simulink model "PILEncoder"  (R2021a)
settings: Solver=FixedStepAuto  StartTime=0.0  StopTime=41.24  FixedStep=0.001  RelTol=1e-3  EnableMultiTasking=on
values from neighbouring files (symbols this model uses):
  den_lpf_d = den_lpf20    [Mainframe_init.m]    (also in load_autopilot.m)
  Emulated_FCC_IO_Delay = 7    [Mainframe_init.m]
  Enable_Gyros = 0    [Mainframe_init.m]
  Enable_INS = 0    [Mainframe_init.m]
  num_lpf_d = num_lpf20    [Mainframe_init.m]    (also in load_autopilot.m)
undefined symbols (not defined in the file or in its folder): act_dmp, act_omega, Actuator, Aerodynamics, aMode, Autopilot, AUX, c_b_WGS, c_be, c_flat, c_grav, c_h_geop0, c_h_geope, c_pa0, c_pe, c_r0, c_rot, c_rsma, c_Tmp0, d_siB_0, d_siB_max, d_siB_min, dd_siB_max, dd_siB_min, dev, DiscIntNeverNeededParam, e_pa, e_Tmp, Earth, fin_maxrate, flag_I_act_switch, flag_I_aero_switch, flag_I_flat, flag_I_gravity_switch, flag_I_rot, Flight_Logic, hcr, HIL_Data, JMMM_0, JMMM_e, JSPB_e, lat_0, lon_0, Main, Mass_Props, mB_0, mM_0, mM_e, pBII_0, pMPB, pNPB, propellant_kg, prp_FBPB, prp_mdot, prp_T, pSPB, pwm_output0, pwm_output1, qEG_0, qIB_0 ... (+30)
libraries: simulink x42, simulink_extras x24, aerolibcommonsys x4, px4lib x2, custom_blocks x1, dspstat3 x1, pil_lib x1, aerolibtransform2 x1, dspnetwork x1, aerolibnav x1
(part 9 of 16)

== system PILEncoder/Non-linear Flight Dynamic Model/GRM_Airframe/stream_flow/calc_stream_flow/velocity_vector_transformation/cross_product ==
  note: Outputs [size]:
      |
      | r1 x r2  [3x1]
  note: Inputs [size]:
      |
      | r1 [3x1]
      | r2 [3x1]
  r1 : Inport
  r2 : Inport  Port=2
  Demux2 : Demux  Outputs=[1;1;1]
      settings: DisplayOption=none
  Demux3 : Demux  Outputs=[1;1;1]
      settings: DisplayOption=none
  Product{2..7} (6 alike) : Product  InputSameDT=on  RndMeth=Zero  SaturateOnIntegerOverflow=on  OutDataTypeStr=Inherit: Same as first input
  Sum : Sum  Inputs=+-  InputSameDT=on  SaturateOnIntegerOverflow=on  OutDataTypeStr=Inherit: Same as first input
  Sum1 : Sum  Inputs=+-  InputSameDT=on  SaturateOnIntegerOverflow=on  OutDataTypeStr=Inherit: Same as first input
  Sum2 : Sum  Inputs=+-  InputSameDT=on  SaturateOnIntegerOverflow=on  OutDataTypeStr=Inherit: Same as first input
  Vector Concatenate : Concatenate  NumInputs=3  Mode=Multidimensional array
  r1_x_r2 : Outport  PortDimensions=[3,1]  VectorParamsAs1DForOutWhenUnconnected=off
  wires:
  Demux2/2 -> Product2/1, Product7/1
  Demux3/3 -> Product5/2, Product2/2
  Demux3/2 -> Product6/2, Product3/2
  Demux2/3 -> Product3/1, Product4/1
  Demux3/1 -> Product7/2, Product4/2
  Demux2/1 -> Product6/1, Product5/1
  Product2/1 -> Sum/1
  Product3/1 -> Sum/2
  Product4/1 -> Sum1/1
  Product5/1 -> Sum1/2
  Product6/1 -> Sum2/1
  Product7/1 -> Sum2/2
  Sum/1 -> Vector Concatenate/1
  Sum1/1 -> Vector Concatenate/2
  Sum2/1 -> Vector Concatenate/3
  r1/1 -> Demux2/1
  r2/1 -> Demux3/1
  Vector Concatenate/1 -> r1_x_r2/1

== system PILEncoder/Non-linear Flight Dynamic Model/GRM_Airframe/weight_and_balance/moi/moi_coordinate_transformation/3_rot_mat ==
  wi1 : Inport
  wi2 : Inport  Port=2
  wi3 : Inport  Port=3
  1. Rotation x-Achse : Subsystem
  1. Rotation y-Achse : Subsystem
  1. Rotation z-Achse : Subsystem
  2. Rotation x-Achse : Subsystem
  2. Rotation y-Achse : Subsystem
  2. Rotation z-Achse : Subsystem
  3. Rotation : Product  Inputs=***  Multiplication=Matrix(*)
  3. Rotation x-Achse : Subsystem
  3. Rotation y-Achse : Subsystem
  3. Rotation z-Achse : Subsystem
  Constant : Constant  Value=rot_1
  Constant1 : Constant  Value=rot_2
  Constant2 : Constant  Value=rot_3
  Multiport Switch : MultiPortSwitch
  Multiport Switch1 : MultiPortSwitch
  Multiport Switch2 : MultiPortSwitch
  T12 : Outport  VectorParamsAs1DForOutWhenUnconnected=off
  wires:
  Multiport Switch2/1 -> 3. Rotation/1
  Multiport Switch1/1 -> 3. Rotation/2
  Multiport Switch/1 -> 3. Rotation/3
  wi3/1 -> 3. Rotation x-Achse/1(alpha3), 3. Rotation z-Achse/1(alpha3), 3. Rotation y-Achse/1(alpha3)
  wi1/1 -> 1. Rotation z-Achse/1(alpha1), 1. Rotation y-Achse/1(alpha1), 1. Rotation x-Achse/1(alpha1)
  wi2/1 -> 2. Rotation z-Achse/1(alpha2), 2. Rotation y-Achse/1(alpha2), 2. Rotation x-Achse/1(alpha2)
  3. Rotation z-Achse/1(3Rot_Matrix_z) -> Multiport Switch2/4
  Constant/1 -> Multiport Switch/1
  1. Rotation x-Achse/1(1Rot_Matrix_x) -> Multiport Switch/2
  Constant1/1 -> Multiport Switch1/1
  1. Rotation y-Achse/1(1Rot_Matrix_y) -> Multiport Switch/3
  1. Rotation z-Achse/1(1Rot_Matrix_z) -> Multiport Switch/4
  Constant2/1 -> Multiport Switch2/1
  3. Rotation/1 -> T12/1  "T12"
  2. Rotation x-Achse/1(2Rot_Matrix_x) -> Multiport Switch1/2
  2. Rotation y-Achse/1(2Rot_Matrix_y) -> Multiport Switch1/3
  2. Rotation z-Achse/1(2Rot_Matrix_z) -> Multiport Switch1/4
  3. Rotation y-Achse/1(3Rot_Matrix_y) -> Multiport Switch2/3
  3. Rotation x-Achse/1(3Rot_Matrix_x) -> Multiport Switch2/2

== system PILEncoder/Non-linear Flight Dynamic Model/GRM_Airframe/weight_and_balance/moi/steiners_theorem_missile/create_deviation_matrix ==
  pBXB : Inport
  Add : Sum
  Add4 : Sum
  Add5 : Sum
  Demux : Demux  Outputs=3
  Gain : Gain  Gain=-1
  Gain1 : Gain  Gain=-1
  Gain3 : Gain  Gain=-1
  Product{1..6} (6 alike) : Product
  Vector Concatenate1 : Concatenate  NumInputs=3  Mode=Multidimensional array  ConcatenateDimension=2
  Vector Concatenate6 : Concatenate  NumInputs=3
  Vector Concatenate7 : Concatenate  NumInputs=3
  Vector Concatenate8 : Concatenate  NumInputs=3
  T_deviation : Outport  VectorParamsAs1DForOutWhenUnconnected=off
  wires:
  Add4/1 -> Vector Concatenate8/3
  Vector Concatenate6/1 -> Vector Concatenate1/1
  Vector Concatenate7/1 -> Vector Concatenate1/2
  Demux/1 -> Product3/1, Product4/1, Product5/2, Product5/1  "a"
  Demux/3 -> Product6/2, Product4/2, Product2/1, Product2/2  "c"
  Gain/1 -> Vector Concatenate7/1, Vector Concatenate6/2
  Gain3/1 -> Vector Concatenate8/2, Vector Concatenate7/3
  Vector Concatenate1/1 -> T_deviation/1
  Demux/2 -> Product3/2, Product1/2, Product1/1, Product6/1  "b"
  Add5/1 -> Vector Concatenate7/2
  Product6/1 -> Gain3/1
  Add/1 -> Vector Concatenate6/1
  Product1/1 -> Add5/1, Add/1
  Product5/1 -> Add4/2, Add5/2
  Product2/1 -> Add4/1, Add/2
  Gain1/1 -> Vector Concatenate8/1, Vector Concatenate6/3
  Product4/1 -> Gain1/1
  Product3/1 -> Gain/1
  Vector Concatenate8/1 -> Vector Concatenate1/3
  pBXB/1 -> Demux/1

== system PILEncoder/Non-linear Flight Dynamic Model/GRM_Airframe/weight_and_balance/moi/steiners_theorem_motor/create_deviation_matrix1 ==
  pBXB : Inport
  Add : Sum
  Add4 : Sum
  Add5 : Sum
  Demux : Demux  Outputs=3
  Gain : Gain  Gain=-1
  Gain1 : Gain  Gain=-1
  Gain3 : Gain  Gain=-1
  Product{1..6} (6 alike) : Product
  Vector Concatenate1 : Concatenate  NumInputs=3  Mode=Multidimensional array  ConcatenateDimension=2
  Vector Concatenate6 : Concatenate  NumInputs=3
  Vector Concatenate7 : Concatenate  NumInputs=3
  Vector Concatenate8 : Concatenate  NumInputs=3
  T_deviation : Outport  VectorParamsAs1DForOutWhenUnconnected=off
  wires:
  pBXB/1 -> Demux/1
  Vector Concatenate8/1 -> Vector Concatenate1/3
  Product3/1 -> Gain/1
  Product4/1 -> Gain1/1
  Gain1/1 -> Vector Concatenate6/3, Vector Concatenate8/1
  Product2/1 -> Add/2, Add4/1
  Product5/1 -> Add5/2, Add4/2
  Product1/1 -> Add/1, Add5/1
  Add/1 -> Vector Concatenate6/1
  Product6/1 -> Gain3/1
  Add5/1 -> Vector Concatenate7/2
  Demux/2 -> Product6/1, Product1/1, Product1/2, Product3/2  "b"
  Vector Concatenate1/1 -> T_deviation/1
  Gain3/1 -> Vector Concatenate7/3, Vector Concatenate8/2
  Gain/1 -> Vector Concatenate6/2, Vector Concatenate7/1
  Demux/3 -> Product2/2, Product2/1, Product4/2, Product6/2  "c"
  Demux/1 -> Product5/1, Product5/2, Product4/1, Product3/1  "a"
  Vector Concatenate7/1 -> Vector Concatenate1/2
  Vector Concatenate6/1 -> Vector Concatenate1/1
  Add4/1 -> Vector Concatenate8/3

== system PILEncoder/Non-linear Flight Dynamic Model/Subsystem1/Extract States/Assemble_States_Bus1/Three-axis Inertial Measurement Unit3/Acceleration Conversion ==
  acceleration : Inport  Unit=m/s^2
  Unit Conversion : UnitConversion
  inherit : Outport  VectorParamsAs1DForOutWhenUnconnected=off
  wires:
  acceleration/1 -> Unit Conversion/1
  Unit Conversion/1 -> inherit/1

== system PILEncoder/Non-linear Flight Dynamic Model/Subsystem1/Extract States/Assemble_States_Bus1/Three-axis Inertial Measurement Unit3/Three-axis Accelerometer ==
  Ab : Inport  Unit=m/s^2  PortDimensions=3
  p q r : Inport  Port=2  Unit=rad/s
  pdot qdot rdot : Inport  Port=3  Unit=rad/s^2
  CG : Inport  Port=4  Unit=m  PortDimensions=3
  g : Inport  Port=5  Unit=m/s^2
  Disallow CGS : UnitConfiguration  UnitSystemsStr=English,SI,SI (extended)  AllowAllUnitSystems=off
  Dynamics : Subsystem
  Gain : Gain  Gain=[1 -1 1]  SaturateOnIntegerOverflow=on  OutDataTypeStr=Inherit: Same as input  ParamDataTypeStr=Inherit: Same as input
  Measurement bias : Constant  Value=a_bias
  Product : Product  Multiplication=Matrix(*)  SaturateOnIntegerOverflow=on  OutDataTypeStr=Inherit: Same as first input
  Random bias : aerolibcommonsys/Tunable White Noise  pwr=a_pow  Ts=0.1  seed=a_seeds
      settings: SourceProductBaseCode=AE
  Reshape1 : Reshape
  Saturation : Saturate  UpperLimit=a_sath  LowerLimit=a_satl
  Scale factors & Cross-coupling errors : Constant  Value=a_sf_cc
  Sum : Sum  Inputs=+-++  SaturateOnIntegerOverflow=on
  Sum1 : Sum  Inputs=|++  SaturateOnIntegerOverflow=on
  Sum4 : Sum  Inputs=++|  SaturateOnIntegerOverflow=on
  Sum7 : Sum  Inputs=|+-  SaturateOnIntegerOverflow=on
  Zero-Order Hold{,1..4} (5 alike) : Gain  SaturateOnIntegerOverflow=on  OutDataTypeStr=Inherit: Same as input  ParamDataTypeStr=Inherit: Same as input
  w x (w x d) : Subsystem
  wdot x d : Subsystem  mask(CrossProduct){aMode=aMode}
      mask help: shared_aeroblks:sharedaeroblkutil:blockCrossProductDesc
      mask init:
      | if aerosharedtest(gcb)
      |     aerosharedicon('shared');
      | else
      |     sharedautoicon('shared');
      | end
      mask Help: eval('if license(''test'',''Aerospace_Blockset'')aerosharedhelp(''threebythree_cross_product'');elseif license(''test'',''Powertrain_Blockset'')sharedautohelp(''threebythree_cross_product'');end')
      mask Display:
      | text(.5,.5,'Cross\nProduct\nC = AxB', ...
      | 	'HorizontalAlignment','Center',...
      | 	'VerticalAlignment','middle')
  wl_ins : Constant  Value=acc
  Ameas : Outport  Unit=m/s^2  PortDimensions=3  VectorParamsAs1DForOutWhenUnconnected=off
  wires:
  Zero-Order Hold4/1 -> Sum7/1
  Zero-Order Hold3/1 -> wdot x d/1(A)
  Zero-Order Hold/1 -> w x (w x d)/1("p q r ")
  Zero-Order Hold2/1 -> Sum/2
  Zero-Order Hold1/1 -> Sum/1
  g/1 -> Zero-Order Hold2/1
  Gain/1 -> wdot x d/2(B), w x (w x d)/2(distance)
  wl_ins/1 -> Sum7/2
  Sum7/1 -> Gain/1
  Dynamics/1("sp_f ") -> Sum1/1
  Sum4/1 -> Dynamics/1(sp_f)
  Sum1/1 -> Saturation/1
  w x (w x d)/1(w x ( w x d)) -> Sum/3
  Ab/1 -> Zero-Order Hold1/1
  Reshape1/1 -> Sum4/1
  Measurement bias/1 -> Sum4/2
  Product/1 -> Reshape1/1
  CG/1 -> Zero-Order Hold4/1
  pdot qdot rdot/1 -> Zero-Order Hold3/1
  p q r/1 -> Zero-Order Hold/1
  Sum/1 -> Product/2
  wdot x d/1(C) -> Sum/4
  Scale factors & Cross-coupling errors/1 -> Product/1
  Random bias/1 -> Sum1/2
  Saturation/1 -> Ameas/1

== system PILEncoder/Non-linear Flight Dynamic Model/Subsystem1/Extract States/Assemble_States_Bus1/Three-axis Inertial Measurement Unit3/Three-axis Gyroscope ==
  p q r : Inport  Unit=rad/s  PortDimensions=3
  G's : Inport  Port=2  Unit=gn  PortDimensions=3
  Disallow CGS : UnitConfiguration  UnitSystemsStr=English,SI,SI (extended)  AllowAllUnitSystems=off
  Dynamics : Subsystem
  Measurement bias : Constant  Value=g_bias
  Product : Product  Multiplication=Matrix(*)  SaturateOnIntegerOverflow=on  OutDataTypeStr=Inherit: Same as first input
  Product1 : Product  SaturateOnIntegerOverflow=on  OutDataTypeStr=Inherit: Same as first input
  Random bias : aerolibcommonsys/Tunable White Noise  pwr=g_pow  Ts=0.1  seed=g_seeds
      settings: SourceProductBaseCode=AE
  Saturation : Saturate  UpperLimit=g_sath  LowerLimit=g_satl
  "Scale factors & Cross-coupling errors " : Constant  Value=g_sf_cc
  Sum1 : Sum  Inputs=|++  SaturateOnIntegerOverflow=on
  Sum4 : Sum  Inputs=+++  SaturateOnIntegerOverflow=on
  Zero-Order Hold : Gain  SaturateOnIntegerOverflow=on  OutDataTypeStr=Inherit: Same as input  ParamDataTypeStr=Inherit: Same as input
  Zero-Order Hold1 : Gain  SaturateOnIntegerOverflow=on  OutDataTypeStr=Inherit: Same as input  ParamDataTypeStr=Inherit: Same as input
  g-sensitive bias : Constant  Value=g_sen
  (p q r)_meas : Outport  Unit=rad/s  PortDimensions=3  VectorParamsAs1DForOutWhenUnconnected=off
  wires:
  Zero-Order Hold1/1 -> Product1/1
  Zero-Order Hold/1 -> Product/2
  Product1/1 -> Sum4/3
  Dynamics/1("p q r ") -> Sum1/1
  G's/1 -> Zero-Order Hold1/1
  Sum1/1 -> Saturation/1
  g-sensitive bias/1 -> Product1/2
  p q r/1 -> Zero-Order Hold/1
  Saturation/1 -> (p q r)_meas/1
  Random bias/1 -> Sum1/2
  "Scale factors & Cross-coupling errors "/1 -> Product/1
  Sum4/1 -> Dynamics/1(p q r)
  Product/1 -> Sum4/1
  Measurement bias/1 -> Sum4/2

== system PILEncoder/Non-linear Flight Dynamic Model/Subsystem1/GRM_Airframe/aerodynamics/aerodynamic_via_lookup/calc_aero_coefficients ==
  dela_deg : Inport
  dele_deg : Inport  Port=2
  delr_deg : Inport  Port=3
  pBIB_star_rps : Inport  Port=4
  qBIB_star_rps : Inport  Port=5
  rBIB_star_rps : Inport  Port=6
  alB_deg : Inport  Port=7
  beB_deg : Inport  Port=8
  CLL_TLU : Subsystem
  CLM_TLU : Subsystem
  CLN_TLU : Subsystem
  CX_TLU : Subsystem
  CY_TLU : Subsystem
  CZ_TLU : Subsystem
  alB_deg D{1..5} (5 alike) : InportShadow  Port=7
  beB_deg D{1..5} (5 alike) : InportShadow  Port=8
  dela_deg D{1..6} (6 alike) : InportShadow
  dele_deg D{1..4} (4 alike) : InportShadow  Port=2
  delr_deg D{1..5} (5 alike) : InportShadow  Port=3
  Cx : Outport  VectorParamsAs1DForOutWhenUnconnected=off
  Cy : Outport  Port=2  VectorParamsAs1DForOutWhenUnconnected=off
  Cz : Outport  Port=3  VectorParamsAs1DForOutWhenUnconnected=off
  Cl : Outport  Port=4  VectorParamsAs1DForOutWhenUnconnected=off
  Cm : Outport  Port=5  VectorParamsAs1DForOutWhenUnconnected=off
  Cn : Outport  Port=6  VectorParamsAs1DForOutWhenUnconnected=off
  wires:
  CX_TLU/1(CX) -> Cx/1
  alB_deg/1 -> CX_TLU/1(alpha_deg)
  beB_deg/1 -> CX_TLU/2(beta_deg)
  dele_deg/1 -> CX_TLU/3(dele_deg)
  dela_deg/1 -> CX_TLU/4(dela_deg)
  CY_TLU/1(CY) -> Cy/1
  beB_deg D1/1 -> CY_TLU/2(beta_deg)
  alB_deg D1/1 -> CY_TLU/1(alpha_deg)
  delr_deg/1 -> CX_TLU/5(delr_deg)
  CZ_TLU/1(CZ) -> Cz/1
  CLL_TLU/1(CLL) -> Cl/1
  CLM_TLU/1(CLM) -> Cm/1
  CLN_TLU/1(CLN) -> Cn/1
  pBIB_star_rps/1 -> CLL_TLU/6(p_ND_rps)
  qBIB_star_rps/1 -> CLM_TLU/6(q_ND_rps)
  rBIB_star_rps/1 -> CLN_TLU/6(r_ND_rps)
  alB_deg D2/1 -> CZ_TLU/1(alpha_deg)
  beB_deg D2/1 -> CZ_TLU/2(beta_deg)
  dele_deg D1/1 -> CY_TLU/3(dele_deg)
  dela_deg D1/1 -> CY_TLU/4(dela_deg)
  delr_deg D1/1 -> CY_TLU/5(delr_deg)
  dele_deg D2/1 -> CZ_TLU/3(dele_deg)
  dela_deg D2/1 -> CZ_TLU/4(dela_deg)
  delr_deg D2/1 -> CZ_TLU/5(delr_deg)
  dela_deg D3/1 -> CLN_TLU/3(dele_deg)
  dela_deg D4/1 -> CLN_TLU/4(dela_deg)
  delr_deg D3/1 -> CLN_TLU/5(delr_deg)
  alB_deg D5/1 -> CLN_TLU/1(alpha_deg)
  alB_deg D4/1 -> CLM_TLU/1(alpha_deg)
  alB_deg D3/1 -> CLL_TLU/1(alpha_deg)
  beB_deg D3/1 -> CLL_TLU/2(beta_deg)
  beB_deg D4/1 -> CLM_TLU/2(beta_deg)
  beB_deg D5/1 -> CLN_TLU/2(beta_deg)
  dele_deg D3/1 -> CLL_TLU/3(dele_deg)
  dele_deg D4/1 -> CLM_TLU/3(dele_deg)
  dela_deg D5/1 -> CLL_TLU/4(dela_deg)
  dela_deg D6/1 -> CLM_TLU/4(dela_deg)
  delr_deg D4/1 -> CLL_TLU/5(delr_deg)
  delr_deg D5/1 -> CLM_TLU/5(delr_deg)

== system PILEncoder/Non-linear Flight Dynamic Model/Subsystem1/GRM_Airframe/aerodynamics/aerodynamic_via_lookup/calc_aero_for_mom ==
  hBE : Inport
  pBPB : Inport  Port=2
  qdynB : Inport  Port=3
  Cx : Inport  Port=4
  Cy : Inport  Port=5
  Cz : Inport  Port=6
  Cl : Inport  Port=7
  Cm : Inport  Port=8
  Cn : Inport  Port=9
  Add : Sum
  Constant1 : Constant  Value=Aerodynamics.lref
      settings: AttributesFormatString=%<Value>
  Constant2 : Constant  Value=Aerodynamics.sref
      settings: AttributesFormatString=%<Value>
  Product : Product
  Product1 : Product  Inputs=3
  Product2 : Product
  Subtract : Sum  Inputs=+-
  Vector Concatenate1 : Concatenate  NumInputs=3
  Vector Concatenate2 : Concatenate  NumInputs=3
  create_pAPB : Subsystem
  cross_product : Subsystem
      mask help: cross product r3 = r1 x r2
      mask Help:
      | Name:
      | 
      |     cross_product
      | 
      | Description:
      | 
      |     This block implements the cross product r3 = r1 x r2.
      | 
      | Inputs  [size] [data type] [unit]:
      | 
      |     vector 1  [3] [double] [-]
      |     vector 2  [3] [double] [-]
      | 
      | Outputs  [size] [data type] [unit]:
      | 
      |     resulting vector  [3] [double] [-]
      mask Display: disp(' r3 = r1 x r2')
  launch_rail : Subsystem
  launch_rail1 : Subsystem
  FBAB : Outport  VectorParamsAs1DForOutWhenUnconnected=off
  MBAB : Outport  Port=2  VectorParamsAs1DForOutWhenUnconnected=off
  wires:
  Cy/1 -> Vector Concatenate2/2
  Cm/1 -> Vector Concatenate1/2
  Cz/1 -> Vector Concatenate2/3
  Cx/1 -> Vector Concatenate2/1
  Cl/1 -> Vector Concatenate1/1
  Cn/1 -> Vector Concatenate1/3
  qdynB/1 -> Product2/2
  Vector Concatenate1/1 -> Product1/2
  Vector Concatenate2/1 -> Product/1
  pBPB/1 -> Subtract/2
  Product/1 -> launch_rail/2(FBAB_c), cross_product/2(r2)  "FBAB"
  Product1/1 -> Add/2  "MBAB"
  Add/1 -> launch_rail1/2(MBAB_c)  "MBAB"
  Constant1/1 -> Product1/3
  Constant2/1 -> Product2/1
  Product2/1 -> Product1/1, Product/2
  cross_product/1(r1_x_r2) -> Add/1
  hBE/1 -> launch_rail1/1(hBE), launch_rail/1(hBE)
  launch_rail1/1(MBAB) -> MBAB/1
  launch_rail/1(FBAB) -> FBAB/1
  Subtract/1 -> cross_product/1(r1)  "pBAB"
  create_pAPB/1(pAPB) -> Subtract/1

== system PILEncoder/Non-linear Flight Dynamic Model/Subsystem1/GRM_Airframe/environment/WGS84_Gravitation/WGS84_2_ECEF ==
  h : Inport
  lon : Inport  Port=2
  lat : Inport  Port=3
  Add1 : Sum  Inputs=+-
  Add2 : Sum
  Add3 : Sum
  Constant : Constant
  Divide : Product  Inputs=***
  Divide1 : Product  Inputs=***
  Divide2 : Product  Inputs=**
  Divide3 : Product  Inputs=**
  Divide4 : Product  Inputs=**
  Mux : Mux  Inputs=3
  Trigonometric Function : Trigonometry
  Trigonometric Function1 : Trigonometry  Operator=cos
  Trigonometric Function2 : Trigonometry
  Trigonometric Function3 : Trigonometry  Operator=cos
  "WGS84 Transformation Parameter " : Subsystem
  pE : Outport  VectorParamsAs1DForOutWhenUnconnected=off
  wires:
  Divide1/1 -> Mux/2  "y_ECEF"
  Add2/1 -> Divide4/1
  Divide/1 -> Mux/1  "x_ECEF"
  lat/1 -> "WGS84 Transformation Parameter "/1(phi), Trigonometric Function3/1, Trigonometric Function2/1
  Divide2/1 -> Add1/2
  Divide3/1 -> Add2/2  "N(1-e^2)"
  Constant/1 -> Add1/1
  Add1/1 -> Divide3/2
  Divide4/1 -> Mux/3  "z_ECEF"
  "WGS84 Transformation Parameter "/1(N) -> Add3/2, Divide3/1
  "WGS84 Transformation Parameter "/2(e) -> Divide2/2, Divide2/1
  h/1 -> Add2/1, Add3/1
  Trigonometric Function1/1 -> Divide/2  "cos(lambda)"
  Trigonometric Function3/1 -> Divide1/3, Divide/3  "cos(phi)"
  Mux/1 -> pE/1  "pE"
  lon/1 -> Trigonometric Function1/1, Trigonometric Function/1
  Add3/1 -> Divide1/1, Divide/1
  Trigonometric Function2/1 -> Divide4/2  "sin(phi)"
  Trigonometric Function/1 -> Divide1/2  "sin(lambda)"

== system PILEncoder/Non-linear Flight Dynamic Model/Subsystem1/GRM_Airframe/environment/atmosphere_static_ISO_2533/density ==
  Tmp : Inport
  pa : Inport  Port=2
  Divide : Product  Inputs=/*/
  specific_gas_constant : Constant  Value=sgc
  rho : Outport  VectorParamsAs1DForOutWhenUnconnected=off
  wires:
  Tmp/1 -> Divide/1
  Divide/1 -> rho/1  "rho"
  pa/1 -> Divide/2
  specific_gas_constant/1 -> Divide/3

== system PILEncoder/Non-linear Flight Dynamic Model/Subsystem1/GRM_Airframe/environment/atmosphere_static_ISO_2533/geopot_height ==
  hBE : Inport
  Add : Sum
  Divide : Product  Inputs=*/*
  mean_earth_radius : Constant  Value=mean_earth_radius
  h_geop : Outport  VectorParamsAs1DForOutWhenUnconnected=off
  wires:
  mean_earth_radius/1 -> Divide/3, Add/2
  Divide/1 -> h_geop/1  "h_geop"
  hBE/1 -> Add/1, Divide/1
  Add/1 -> Divide/2

== system PILEncoder/Non-linear Flight Dynamic Model/Subsystem1/GRM_Airframe/environment/atmosphere_static_ISO_2533/speed_of_sound ==
  Tmp : Inport
  Product : Product  Inputs=3
  Sqrt : Sqrt  SaturateOnIntegerOverflow=on
  heat_capacity_ratio : Constant  Value=hcr
  specific_gas_constant : Constant  Value=sgc
  sos : Outport  VectorParamsAs1DForOutWhenUnconnected=off
  wires:
  Sqrt/1 -> sos/1  "sos"
  Tmp/1 -> Product/3
  Product/1 -> Sqrt/1
  heat_capacity_ratio/1 -> Product/2
  specific_gas_constant/1 -> Product/1

== system PILEncoder/Non-linear Flight Dynamic Model/Subsystem1/GRM_Airframe/environment/atmosphere_static_ISO_2533/tmp_and_pressure_ISO_2533 ==
  h_geop : Inport
  e_Tmp : Inport  Port=2
  e_pa : Inport  Port=3
  Subtract1 : Sum
  Subtract2 : Sum
  Tmp_norm_msl : Constant  Value=c_Tmp0
  geopotential_height_ref : Constant  Value=c_h_geop0
  pa_norm_msl : Constant  Value=c_pa0
  static_Temperature : Subsystem
  static_pressure : Subsystem
  Tmp : Outport  VectorParamsAs1DForOutWhenUnconnected=off
  pa : Outport  Port=2  VectorParamsAs1DForOutWhenUnconnected=off
  wires:
  h_geop/1 -> static_pressure/2(h_geop), static_Temperature/2(h_geop)
  Subtract2/1 -> static_pressure/4(pa_ref)  "pa_ref"
  pa_norm_msl/1 -> Subtract2/2
  Subtract1/1 -> static_pressure/3(Tmp_ref), static_Temperature/1(Tmp_ref)  "Tmp_ref"
  static_pressure/1(pa) -> pa/1
  e_pa/1 -> Subtract2/1
  static_Temperature/1(Tmp) -> Tmp/1
  e_Tmp/1 -> Subtract1/1
  geopotential_height_ref/1 -> static_pressure/1(h_geop_ref), static_Temperature/3(h_geop_ref)  "h_geop_ref"
  Tmp_norm_msl/1 -> Subtract1/2

== system PILEncoder/Non-linear Flight Dynamic Model/Subsystem1/GRM_Airframe/gravity/launch_rail/initial_altitude ==
  Constant : Constant  Value=pBII_0
  Constant2 : Constant  Value=flag_I_flat
  Demux : Demux  Outputs=3
  Gain : Gain  Gain=-1
  Switch1 : Switch  Criteria=u2 > Threshold
  Terminator{,1..3} (4 alike) : Terminator
  trafo_E_to_geodetic : Subsystem  mask(Transformation der ECEF Position in geodätische Größen){}
      mask help: Dieser Block transformiert die Position im ECEF KOS in die geodätische Länge, Breite und Höhe
      mask init:
      | [c_mue, c_rsma, c_flat] = init_transformations_earth;
      mask Help:
      | Name:
      | 
      |     trafo_E_to_geodetic
      | 
      | Beschreibung:
      | 
      |     Dieser Block transformiert die Position im ECEF KOS in die geodätische
      |     Länge, Breite und Höhe.
      | 
      | Inputs   [size]  [data type] [unit]:
      | 
      |     pBEE    [3] [double] [m]
      | 
      | Outputs  [size]  [data type] [unit]:
      | 
      |     long  [1] [double] [rad]
      |     lat   [1] [double] [rad]
      |     alt   [1] [double] [m]
      | 
      | Parameter
      | 
      |    c_rsma
      |    c_flat
  hBE_0 : Outport  VectorParamsAs1DForOutWhenUnconnected=off
  wires:
  Constant2/1 -> Switch1/2
  trafo_E_to_geodetic/3(alt) -> Switch1/3  "hBE_0"
  Demux/2 -> Terminator3/1
  Demux/3 -> Gain/1
  Gain/1 -> Switch1/1
  Demux/1 -> Terminator2/1
  trafo_E_to_geodetic/2(lat) -> Terminator1/1
  Constant/1 -> Demux/1, trafo_E_to_geodetic/1(pBEE)
  trafo_E_to_geodetic/1(lon) -> Terminator/1
  Switch1/1 -> hBE_0/1  "hBE_0"

== system PILEncoder/Non-linear Flight Dynamic Model/Subsystem1/GRM_Airframe/motion_kinematics/calc_motion_kinematics/calc_transformation_matrix ==
  qIE : Inport
  qEG : Inport  Port=2
  qIB : Inport  Port=3
  T12_from_q1 : Subsystem
      mask help: Transforms a quaternion into a Direction Cosine Matrix
      mask Help:
      | Name:
      | 
      |     T12_from_q12
      | 
      | Description:
      | 
      |     This block implements the transformation of a quaternion into the
      |     corresponding direction cosine matrix DCM.
      | 
      | Inputs  [size] [data type] [unit]:
      | 
      |     quaternion q12 [4] [double] [-]
      | 
      | Outputs  [size] [data type] [unit]:
      | 
      |     direction cosine matrix T12  [3x3] [double] [-]
      mask Display:
      | %port_label('input', 1, 'q12')
      | %port_label('output', 1, 'T12')
      | disp('q \rightarrow DCM','texmode','on')
  T12_from_q12 : Subsystem
      mask help: Transforms a quaternion into a Direction Cosine Matrix
      mask Help:
      | Name:
      | 
      |     T12_from_q12
      | 
      | Description:
      | 
      |     This block implements the transformation of a quaternion into the
      |     corresponding direction cosine matrix DCM.
      | 
      | Inputs  [size] [data type] [unit]:
      | 
      |     quaternion q12 [4] [double] [-]
      | 
      | Outputs  [size] [data type] [unit]:
      | 
      |     direction cosine matrix T12  [3x3] [double] [-]
      mask Display:
      | %port_label('input', 1, 'q12')
      | %port_label('output', 1, 'T12')
      | disp('q \rightarrow DCM','texmode','on')
  T12_from_q2 : Subsystem
      mask help: Transforms a quaternion into a Direction Cosine Matrix
      mask Help:
      | Name:
      | 
      |     T12_from_q12
      | 
      | Description:
      | 
      |     This block implements the transformation of a quaternion into the
      |     corresponding direction cosine matrix DCM.
      | 
      | Inputs  [size] [data type] [unit]:
      | 
      |     quaternion q12 [4] [double] [-]
      | 
      | Outputs  [size] [data type] [unit]:
      | 
      |     direction cosine matrix T12  [3x3] [double] [-]
      mask Display:
      | %port_label('input', 1, 'q12')
      | %port_label('output', 1, 'T12')
      | disp('q \rightarrow DCM','texmode','on')
  conjugate_quaternion : Subsystem
      mask help: conjugate a quaternion
      mask Help:
      | Name:
      | 
      |     conjugate_quaternion
      | 
      | Description:
      | 
      |     computes the conjugate quaternion
      | 
      | Inputs  [size] [data type] [unit]:
      | 
      |     quaternion q_2_1  [4] [double] [-]
      | 
      | Outputs  [size] [data type] [unit]:
      | 
      |     conjugated quaternion q_1_2  [4] [double] [-]
      mask Display: disp (' conj(q)')
  q31_from_q32_mul_q1 : Subsystem
      mask help: multiply two quaternions
      mask Help:
      | Name:
      | 
      |     q31_from_q32_mul_q21
      | 
      | Description:
      | 
      |     This block implements the multiplication of two quaternions according
      |     to q31=q32*q21.
      | 
      | Inputs  [size] [data type] [unit]:
      | 
      |     attitude quaternion q32  [4] [double] [-]
      |     attitude quaternion q21  [4] [double] [-]
      | 
      | Outputs  [size] [data type] [unit]:
      | 
      |     attitude quaternion q31  [4] [double] [-]
      mask Display:
      | port_label('input', 1, 'q32')
      | port_label('input', 2, 'q21')
      | port_label('output', 1, 'q31')
      | disp('q_{31} = q_{32} {\bf\cdot} q_{21}','texmode','on')
  q31_from_q32_mul_q2 : Subsystem
      mask help: multiply two quaternions
      mask Help:
      | Name:
      | 
      |     q31_from_q32_mul_q21
      | 
      | Description:
      | 
      |     This block implements the multiplication of two quaternions according
      |     to q31=q32*q21.
      | 
      | Inputs  [size] [data type] [unit]:
      | 
      |     attitude quaternion q32  [4] [double] [-]
      |     attitude quaternion q21  [4] [double] [-]
      | 
      | Outputs  [size] [data type] [unit]:
      | 
      |     attitude quaternion q31  [4] [double] [-]
      mask Display:
      | port_label('input', 1, 'q32')
      | port_label('input', 2, 'q21')
      | port_label('output', 1, 'q31')
      | disp('q_{31} = q_{32} {\bf\cdot} q_{21}','texmode','on')
  q31_from_q32_mul_q21 : Subsystem
      mask help: multiply two quaternions
      mask Help:
      | Name:
      | 
      |     q31_from_q32_mul_q21
      | 
      | Description:
      | 
      |     This block implements the multiplication of two quaternions according
      |     to q31=q32*q21.
      | 
      | Inputs  [size] [data type] [unit]:
      | 
      |     attitude quaternion q32  [4] [double] [-]
      |     attitude quaternion q21  [4] [double] [-]
      | 
      | Outputs  [size] [data type] [unit]:
      | 
      |     attitude quaternion q31  [4] [double] [-]
      mask Display:
      | port_label('input', 1, 'q32')
      | port_label('input', 2, 'q21')
      | port_label('output', 1, 'q31')
      | disp('q_{31} = q_{32} {\bf\cdot} q_{21}','texmode','on')
  TEB : Outport  VectorParamsAs1DForOutWhenUnconnected=off
  TGB : Outport  Port=2  VectorParamsAs1DForOutWhenUnconnected=off
  TIB : Outport  Port=3  VectorParamsAs1DForOutWhenUnconnected=off
  wires:
  T12_from_q2/1(T12) -> TGB/1  "TGB"
  q31_from_q32_mul_q21/1(q31) -> conjugate_quaternion/1(q)  "qIG"
  qIB/1 -> q31_from_q32_mul_q1/2(q21), T12_from_q12/1(q12)
  q31_from_q32_mul_q1/1(q31) -> T12_from_q2/1(q12), q31_from_q32_mul_q2/2(q21)  "qGB"
  qEG/1 -> q31_from_q32_mul_q21/2(q21), q31_from_q32_mul_q2/1(q32)
  T12_from_q1/1(T12) -> TEB/1  "TEB"
  conjugate_quaternion/1(q_conj) -> q31_from_q32_mul_q1/1(q32)  "qGI"
  qIE/1 -> q31_from_q32_mul_q21/1(q32)
  q31_from_q32_mul_q2/1(q31) -> T12_from_q1/1(q12)  "qEB"
  T12_from_q12/1(T12) -> TIB/1  "TIB"

== system PILEncoder/Non-linear Flight Dynamic Model/Subsystem1/GRM_Airframe/motion_kinematics/calc_motion_kinematics/earth_rotation ==
  lat : Inport
  lon : Inport  Port=2
  Gain : Gain
  Gain1 : Gain
  earth_rotation_rate : Subsystem
  quaternion_integration : Subsystem
  quaternion_integration1 : Subsystem
  transport_rate : Subsystem
  wIEE : Outport  VectorParamsAs1DForOutWhenUnconnected=off
  TIE : Outport  Port=2  VectorParamsAs1DForOutWhenUnconnected=off
  qIE : Outport  Port=3  VectorParamsAs1DForOutWhenUnconnected=off
  qEG : Outport  Port=4  VectorParamsAs1DForOutWhenUnconnected=off
  TEG : Outport  Port=5  VectorParamsAs1DForOutWhenUnconnected=off
  wEGG : Outport  Port=6  VectorParamsAs1DForOutWhenUnconnected=off
  wires:
  earth_rotation_rate/1(wIEE) -> wIEE/1, Gain/1
  Gain/1 -> quaternion_integration/1(wEIE)  "wEIE"
  quaternion_integration/1(qIE) -> qIE/1
  quaternion_integration/2(TIE) -> TIE/1
  lat/1 -> transport_rate/1(lat)
  lon/1 -> transport_rate/2(lon)
  transport_rate/1(wEGG) -> wEGG/1, Gain1/1
  Gain1/1 -> quaternion_integration1/1(wGEG)  "wGEG"
  quaternion_integration1/1(qEG) -> qEG/1
  quaternion_integration1/2(TEG) -> TEG/1

== system PILEncoder/Non-linear Flight Dynamic Model/Subsystem1/GRM_Airframe/propulsion/prp_uncertainty/3_rot_mat ==
  wi1 : Inport
  wi2 : Inport  Port=2
  wi3 : Inport  Port=3
  1. Rotation x-Achse : Subsystem
  1. Rotation y-Achse : Subsystem
  1. Rotation z-Achse : Subsystem
  2. Rotation x-Achse : Subsystem
  2. Rotation y-Achse : Subsystem
  2. Rotation z-Achse : Subsystem
  3. Rotation : Product  Inputs=***  Multiplication=Matrix(*)
  3. Rotation x-Achse : Subsystem
  3. Rotation y-Achse : Subsystem
  3. Rotation z-Achse : Subsystem
  Constant : Constant  Value=rot_1
  Constant1 : Constant  Value=rot_2
  Constant2 : Constant  Value=rot_3
  Multiport Switch : MultiPortSwitch
  Multiport Switch1 : MultiPortSwitch
  Multiport Switch2 : MultiPortSwitch
  T12 : Outport  VectorParamsAs1DForOutWhenUnconnected=off
  wires:
  Multiport Switch2/1 -> 3. Rotation/1
  Multiport Switch1/1 -> 3. Rotation/2
  Multiport Switch/1 -> 3. Rotation/3
  wi3/1 -> 3. Rotation x-Achse/1(alpha3), 3. Rotation z-Achse/1(alpha3), 3. Rotation y-Achse/1(alpha3)
  wi1/1 -> 1. Rotation z-Achse/1(alpha1), 1. Rotation y-Achse/1(alpha1), 1. Rotation x-Achse/1(alpha1)
  wi2/1 -> 2. Rotation z-Achse/1(alpha2), 2. Rotation y-Achse/1(alpha2), 2. Rotation x-Achse/1(alpha2)
  3. Rotation z-Achse/1(3Rot_Matrix_z) -> Multiport Switch2/4
  Constant/1 -> Multiport Switch/1
  1. Rotation x-Achse/1(1Rot_Matrix_x) -> Multiport Switch/2
  Constant1/1 -> Multiport Switch1/1
  1. Rotation y-Achse/1(1Rot_Matrix_y) -> Multiport Switch/3
  1. Rotation z-Achse/1(1Rot_Matrix_z) -> Multiport Switch/4
  Constant2/1 -> Multiport Switch2/1
  3. Rotation/1 -> T12/1  "T12"
  2. Rotation x-Achse/1(2Rot_Matrix_x) -> Multiport Switch1/2
  2. Rotation y-Achse/1(2Rot_Matrix_y) -> Multiport Switch1/3
  2. Rotation z-Achse/1(2Rot_Matrix_z) -> Multiport Switch1/4
  3. Rotation y-Achse/1(3Rot_Matrix_y) -> Multiport Switch2/3
  3. Rotation x-Achse/1(3Rot_Matrix_x) -> Multiport Switch2/2

== system PILEncoder/Non-linear Flight Dynamic Model/Subsystem1/GRM_Airframe/propulsion/prp_uncertainty/cross_product ==
  note: Outputs [size]:
      |
      | r1 x r2  [3x1]
  note: Inputs [size]:
      |
      | r1 [3x1]
      | r2 [3x1]
  r1 : Inport
  r2 : Inport  Port=2
  Demux2 : Demux  Outputs=[1;1;1]
      settings: DisplayOption=none
  Demux3 : Demux  Outputs=[1;1;1]
      settings: DisplayOption=none
  Product{2..7} (6 alike) : Product  InputSameDT=on  RndMeth=Zero  SaturateOnIntegerOverflow=on  OutDataTypeStr=Inherit: Same as first input
  Sum : Sum  Inputs=+-  InputSameDT=on  SaturateOnIntegerOverflow=on  OutDataTypeStr=Inherit: Same as first input
  Sum1 : Sum  Inputs=+-  InputSameDT=on  SaturateOnIntegerOverflow=on  OutDataTypeStr=Inherit: Same as first input
  Sum2 : Sum  Inputs=+-  InputSameDT=on  SaturateOnIntegerOverflow=on  OutDataTypeStr=Inherit: Same as first input
  Vector Concatenate : Concatenate  NumInputs=3  Mode=Multidimensional array
  r1_x_r2 : Outport  PortDimensions=[3,1]  VectorParamsAs1DForOutWhenUnconnected=off
  wires:
  Demux2/2 -> Product2/1, Product7/1
  Demux3/3 -> Product5/2, Product2/2
  Demux3/2 -> Product6/2, Product3/2
  Demux2/3 -> Product3/1, Product4/1
  Demux3/1 -> Product7/2, Product4/2
  Demux2/1 -> Product6/1, Product5/1
  Product2/1 -> Sum/1
  Product3/1 -> Sum/2
  Product4/1 -> Sum1/1
  Product5/1 -> Sum1/2
  Product6/1 -> Sum2/1
  Product7/1 -> Sum2/2
  Sum/1 -> Vector Concatenate/1
  Sum1/1 -> Vector Concatenate/2
  Sum2/1 -> Vector Concatenate/3
  r1/1 -> Demux2/1
  r2/1 -> Demux3/1
  Vector Concatenate/1 -> r1_x_r2/1

== system PILEncoder/Non-linear Flight Dynamic Model/Subsystem1/GRM_Airframe/rb_eom/calc_bus_flight_dyn_bus_entries/Subsystem2 ==
  TIE : Inport
  pBII : Inport  Port=2
  Constant : Constant  Value=lon_0
  Constant1 : Constant  Value=flag_I_flat
  Constant2 : Constant  Value=lat_0
  Demux : Demux  Outputs=3
  Demux1 : Demux  Outputs=3
  Gain : Gain  Gain=-1
  Math Function : Math  Operator=transpose  SignedPower=on  SaturateOnIntegerOverflow=on
  Product : Product  Multiplication=Matrix(*)
  Switch : Switch  Criteria=u2 > Threshold
  Terminator : Terminator
  Terminator1 : Terminator
  Vector Concatenate : Concatenate  NumInputs=3
  Vector Concatenate1 : Concatenate  NumInputs=3
  trafo_E_to_geodetic : Subsystem  mask(Transformation der ECEF Position in geodätische Größen){}
      mask help: Dieser Block transformiert die Position im ECEF KOS in die geodätische Länge, Breite und Höhe
      mask init:
      | [c_mue, c_rsma, c_flat] = init_transformations_earth;
      mask Help:
      | Name:
      | 
      |     trafo_E_to_geodetic
      | 
      | Beschreibung:
      | 
      |     Dieser Block transformiert die Position im ECEF KOS in die geodätische
      |     Länge, Breite und Höhe.
      | 
      | Inputs   [size]  [data type] [unit]:
      | 
      |     pBEE    [3] [double] [m]
      | 
      | Outputs  [size]  [data type] [unit]:
      | 
      |     long  [1] [double] [rad]
      |     lat   [1] [double] [rad]
      |     alt   [1] [double] [m]
      | 
      | Parameter
      | 
      |    c_rsma
      |    c_flat
  lon : Outport  VectorParamsAs1DForOutWhenUnconnected=off
  lat : Outport  Port=2  VectorParamsAs1DForOutWhenUnconnected=off
  hBE : Outport  Port=3  VectorParamsAs1DForOutWhenUnconnected=off
  wires:
  Demux1/2 -> lat/1  "lat"
  pBII/1 -> Demux/1, Product/2
  Product/1 -> trafo_E_to_geodetic/1(pBEE)  "pBEE"
  Demux1/1 -> lon/1  "lon"
  Demux1/3 -> hBE/1  "hBE"
  trafo_E_to_geodetic/1(lon) -> Vector Concatenate/1  "lon"
  trafo_E_to_geodetic/2(lat) -> Vector Concatenate/2  "lat"
  trafo_E_to_geodetic/3(alt) -> Vector Concatenate/3  "alt"
  Demux/1 -> Terminator/1
  Demux/2 -> Terminator1/1
  Demux/3 -> Gain/1
  Gain/1 -> Vector Concatenate1/3
  Constant/1 -> Vector Concatenate1/1
  Constant2/1 -> Vector Concatenate1/2
  Vector Concatenate/1 -> Switch/3
  Constant1/1 -> Switch/2
  Vector Concatenate1/1 -> Switch/1
  Switch/1 -> Demux1/1
  TIE/1 -> Math Function/1
  Math Function/1 -> Product/1  "TEI"

== system PILEncoder/Non-linear Flight Dynamic Model/Subsystem1/GRM_Airframe/rb_eom/calc_bus_flight_dyn_bus_entries/q12_from_T12 ==
  note: Outputs [size]:
      |
      | quaternion q12 [4x1]
  note: Inputs [size]:
      |
      | direction cosine matrix T12 [3x3]
  T12 : Inport  PortDimensions=[3 3]
  Case 0 : Subsystem
  Case 1 : Subsystem
  Case 2 : Subsystem
  Case 3 : Subsystem
  Constant : Constant
  Constant1 : Constant  Value=-1
  Display{,1..3} (4 alike) : Display
  Merge : Merge  Inputs=4
  Product4 : Product
  Selector : Selector  IndexMode=Zero-based  InputPortWidth=4  IndexOptions=Index vector (dialog)  Indices=3  OutputSizes=1
  Switch : Switch
  dcm11 : Selector  NumberOfDimensions=2  IndexMode=Zero-based  InputPortWidth=3  IndexOptions=Index vector (dialog),Index vector (dialog)  Indices=0,0  OutputSizes=1,1
  dcm22 : Selector  NumberOfDimensions=2  IndexMode=Zero-based  InputPortWidth=3  IndexOptions=Index vector (dialog),Index vector (dialog)  Indices=1,1  OutputSizes=1,1
  dcm33 : Selector  NumberOfDimensions=2  IndexMode=Zero-based  InputPortWidth=3  IndexOptions=Index vector (dialog),Index vector (dialog)  Indices=2,2  OutputSizes=1,1
  normalize_quaternion : Subsystem
      mask help: normalize a quaternion
      mask Help:
      | Name:
      | 
      |     normalize_quaternion
      | 
      | Description:
      | 
      |     This block normalizes the quaternion q21. It should be used as a
      |     safety measure when computing quaternions.
      | 
      | Inputs  [size] [data type] [unit]:
      | 
      |     attitude quaternion q21  [4] [double] [-]
      | 
      | Outputs  [size] [data type] [unit]:
      | 
      |     normalized attitude quaternion q21  [4] [double] [-]
      mask Display: disp (' norm(q)')
  q_R^0(R) : Subsystem  TreatAsAtomicUnit=on
  q_R^1(R) : Subsystem  TreatAsAtomicUnit=on
  q_R^2(R) : Subsystem  TreatAsAtomicUnit=on
  q_R^3(R) : Subsystem  TreatAsAtomicUnit=on
  q12 : Outport  PortDimensions=[4 1]  VectorParamsAs1DForOutWhenUnconnected=off
  wires:
  Constant1/1 -> Switch/3
  Switch/1 -> Product4/2
  Selector/1 -> Switch/2
  normalize_quaternion/1(q_normalized) -> Selector/1, Product4/1
  Constant/1 -> Switch/1
  Product4/1 -> q12/1
  Merge/1 -> normalize_quaternion/1(q)
  q_R^1(R)/1(q_R^1(R)) -> Merge/2
  q_R^2(R)/1(q_R^2(R)) -> Merge/3
  q_R^3(R)/1(q_R^3(R)) -> Merge/4
  q_R^0(R)/1(q_R^0(R)) -> Merge/1
  Case 3/1(q_R^3(R)) -> q_R^3(R)/Enable, Display3/1
  Case 2/1(q_R^2(R)) -> q_R^2(R)/Enable, Display2/1
  T12/1 -> q_R^0(R)/1(DCM), q_R^1(R)/1(DCM), q_R^2(R)/1(DCM), q_R^3(R)/1(DCM), dcm33/1, dcm22/1, dcm11/1
  Case 1/1(q_R^1(R)) -> q_R^1(R)/Enable, Display1/1
  Case 0/1(q_R^0(R)) -> q_R^0(R)/Enable, Display/1
  dcm33/1 -> Case 3/3(dcm33), Case 2/3(dcm33), Case 1/3(dcm33), Case 0/3(dcm33)  "dcm33"
  dcm22/1 -> Case 3/2(dcm22), Case 2/2(dcm22), Case 1/2(dcm22), Case 0/2(dcm22)  "dcm22"
  dcm11/1 -> Case 3/1(dcm11), Case 2/1(dcm11), Case 1/1(dcm11), Case 0/1(dcm11)  "dcm11"

== system PILEncoder/Non-linear Flight Dynamic Model/Subsystem1/GRM_Airframe/rb_eom/calc_bus_flight_dyn_bus_entries/quaternion_to_euler_angles ==
  note: Inputs [size]:
      |
      | quaternion [4]
  note: Outputs [size]:
      |
      | roll angle [1]
      | pitch angle [1]
      | yaw angle [1]
  note: Um numerische Probleme zu
      | vermeiden, wird hier eine Saturiierung
      | benutzt.
  q : Inport  PortDimensions=4
  Add : Sum
  Add1 : Sum  Inputs=+--
  Add2 : Sum  Inputs=+-
  Add3 : Sum
  Add4 : Sum  Inputs=+--
  Complex to Real-Imag : ComplexToRealImag  Output=Real
  Constant : Constant  Value=0.5
  Constant1 : Constant  Value=0.5
  Demux : Demux
  Gain : Gain  Gain=2
  Product{,1..9} (10 alike) : Product
  Saturation : Saturate  UpperLimit=1  LowerLimit=-1
      settings: AttributesFormatString=|
      | %<UpperLimit>
      | %<LowerLimit>
  Trigonometric Function : Trigonometry  Operator=atan2
  Trigonometric Function1 : Trigonometry  Operator=asin
  Trigonometric Function2 : Trigonometry  Operator=atan2
  Vector Concatenate : Concatenate  NumInputs=3
  eulx : Outport  VectorParamsAs1DForOutWhenUnconnected=off
  wires:
  Saturation/1 -> Trigonometric Function1/1
  Gain/1 -> Saturation/1
  Demux/3 -> Product5/2, Product1/2, Product7/1, Product9/1, Product9/2  "3"
  Constant1/1 -> Add4/1
  Product8/1 -> Add4/2
  Product9/1 -> Add4/3
  Constant/1 -> Add1/1
  Demux/2 -> Product6/2, Product8/1, Product8/2, Product1/1, Product3/1, Product3/2, Product4/1  "2"
  Demux/1 -> Product5/1, Product6/1, Product/1, Product2/1, Product2/2  "1"
  Demux/4 -> Product/2, Product4/2, Product7/2  "4"
  q/1 -> Demux/1
  Add1/1 -> Trigonometric Function/2
  Add2/1 -> Gain/1
  Add4/1 -> Trigonometric Function2/2
  Add3/1 -> Trigonometric Function2/1
  Product6/1 -> Add3/1
  Product7/1 -> Add3/2
  Product4/1 -> Add2/1
  Product5/1 -> Add2/2
  Product2/1 -> Add1/2
  Product3/1 -> Add1/3
  Product/1 -> Add/1
  Product1/1 -> Add/2
  Add/1 -> Trigonometric Function/1
  Trigonometric Function/1 -> Vector Concatenate/1
  Trigonometric Function1/1 -> Vector Concatenate/2
  Trigonometric Function2/1 -> Vector Concatenate/3
  Complex to Real-Imag/1 -> eulx/1
  Vector Concatenate/1 -> Complex to Real-Imag/1

== system PILEncoder/Non-linear Flight Dynamic Model/Subsystem1/GRM_Airframe/rb_eom/calc_bus_flight_dyn_bus_entries/quaternion_to_euler_angles1 ==
  note: Um numerische Probleme zu
      | vermeiden, wird hier eine Saturiierung
      | benutzt.
  note: Outputs [size]:
      |
      | roll angle [1]
      | pitch angle [1]
      | yaw angle [1]
  note: Inputs [size]:
      |
      | quaternion [4]
  q : Inport  PortDimensions=4
  Add : Sum
  Add1 : Sum  Inputs=+--
  Add2 : Sum  Inputs=+-
  Add3 : Sum
  Add4 : Sum  Inputs=+--
  Complex to Real-Imag : ComplexToRealImag  Output=Real
  Constant : Constant  Value=0.5
  Constant1 : Constant  Value=0.5
  Demux : Demux
  Gain : Gain  Gain=2
  Product{,1..9} (10 alike) : Product
  Saturation : Saturate  UpperLimit=1  LowerLimit=-1
      settings: AttributesFormatString=|
      | %<UpperLimit>
      | %<LowerLimit>
  Trigonometric Function : Trigonometry  Operator=atan2
  Trigonometric Function1 : Trigonometry  Operator=asin
  Trigonometric Function2 : Trigonometry  Operator=atan2
  Vector Concatenate : Concatenate  NumInputs=3
  eulx : Outport  VectorParamsAs1DForOutWhenUnconnected=off
  wires:
  Vector Concatenate/1 -> Complex to Real-Imag/1
  Complex to Real-Imag/1 -> eulx/1
  Trigonometric Function2/1 -> Vector Concatenate/3
  Trigonometric Function1/1 -> Vector Concatenate/2
  Trigonometric Function/1 -> Vector Concatenate/1
  Add/1 -> Trigonometric Function/1
  Product1/1 -> Add/2
  Product/1 -> Add/1
  Product3/1 -> Add1/3
  Product2/1 -> Add1/2
  Product5/1 -> Add2/2
  Product4/1 -> Add2/1
  Product7/1 -> Add3/2
  Product6/1 -> Add3/1
  Add3/1 -> Trigonometric Function2/1
  Add4/1 -> Trigonometric Function2/2
  Add2/1 -> Gain/1
  Add1/1 -> Trigonometric Function/2
  q/1 -> Demux/1
  Demux/4 -> Product7/2, Product4/2, Product/2  "4"
  Demux/1 -> Product2/2, Product2/1, Product/1, Product6/1, Product5/1  "1"
  Demux/2 -> Product4/1, Product3/2, Product3/1, Product1/1, Product8/2, Product8/1, Product6/2  "2"
  Constant/1 -> Add1/1
  Product9/1 -> Add4/3
  Product8/1 -> Add4/2
  Constant1/1 -> Add4/1
  Demux/3 -> Product9/2, Product9/1, Product7/1, Product1/2, Product5/2  "3"
  Gain/1 -> Saturation/1
  Saturation/1 -> Trigonometric Function1/1

== system PILEncoder/Non-linear Flight Dynamic Model/Subsystem1/GRM_Airframe/rb_eom/eom_6dof/Rigid_Body_EOM_6_DOF ==
  FBTX : Inport  PortDimensions=[3,1]
  MBTB : Inport  Port=2  PortDimensions=[3,1]
  mB : Inport  Port=3  PortDimensions=[1]
  x0 : Inport  Port=4
  JBB : Inport  Port=5  PortDimensions=[3,3]
  d_JBB : Inport  Port=6  PortDimensions=[3,3]
  Bus Selector : BusSelector  OutputSignals=qIB,vBII,wBIB
  Constant : Constant  Value=flag_Kraft
  Integration : Subsystem
  Math Function2 : Math  Operator=transpose  SignedPower=on  SaturateOnIntegerOverflow=on
  Product2 : Product  Multiplication=Matrix(*)
  Switch : Switch  Criteria=u2 > Threshold  Threshold=1
  T12_from_q12 : Subsystem
      mask help: Transforms a quaternion into a Direction Cosine Matrix
      mask Help:
      | Name:
      | 
      |     T12_from_q12
      | 
      | Description:
      | 
      |     This block implements the transformation of a quaternion into the
      |     corresponding direction cosine matrix DCM.
      | 
      | Inputs  [size] [data type] [unit]:
      | 
      |     quaternion q12 [4] [double] [-]
      | 
      | Outputs  [size] [data type] [unit]:
      | 
      |     direction cosine matrix T12  [3x3] [double] [-]
      mask Display:
      | %port_label('input', 1, 'q12')
      | %port_label('output', 1, 'T12')
      | disp('q \rightarrow DCM','texmode','on')
  rb_eom_6dof : Subsystem
  rb_eom : Outport  VectorParamsAs1DForOutWhenUnconnected=off
  wires:
  rb_eom_6dof/4(d_wBIB) -> Integration/4(d_wBIB)  "d_wBIB"
  JBB/1 -> rb_eom_6dof/3(JBB)
  d_JBB/1 -> rb_eom_6dof/5(d_JBB)
  mB/1 -> rb_eom_6dof/2(mB)
  MBTB/1 -> rb_eom_6dof/4(MBTB)
  Switch/1 -> rb_eom_6dof/1(FBTB)
  Constant/1 -> Switch/2
  Product2/1 -> Switch/3
  FBTX/1 -> Product2/2, Switch/1
  Math Function2/1 -> Product2/1
  T12_from_q12/1(T12) -> Math Function2/1
  Bus Selector/2 -> rb_eom_6dof/7(vBII)  "<vBII>"
  x0/1 -> Integration/5(x0)
  Bus Selector/1 -> rb_eom_6dof/6(qIB), T12_from_q12/1(q12)  "<qIB>"
  Bus Selector/3 -> rb_eom_6dof/8(wBIB)  "<wBIB>"
  rb_eom_6dof/1(d_pBII) -> Integration/1(d_pBII)  "d_pBII"
  rb_eom_6dof/2(d_vBII) -> Integration/2(d_vBII)  "d_vBII"
  rb_eom_6dof/3(d_qIB) -> Integration/3(d_qIB)  "d_qIB"
  Integration/1(eom) -> Bus Selector/1, rb_eom/1

== system PILEncoder/Non-linear Flight Dynamic Model/Subsystem1/GRM_Airframe/stream_flow/calc_stream_flow/Subsystem1 ==
  vBEB : Inport
  wBIB : Inport  Port=2
  rho : Inport  Port=3
  sos : Inport  Port=4
  AoA_Sideslip_Alphatot_Phi : Subsystem
      mask help:
      | Aus den Komponenten der Geschwindigkeit im ECEF-System, dargestellt im Body-System vBEB
      | werden Anstellwinkel (alpha), Schiebewinkel (beta), totaler Anstellwinkel (alpha_T) sowie Rollwinkel (phi) berechnet.
      | Die Ausgabe erfolgt als Bus in [rad]
      mask Help:
      | Name:
      | 
      |    AoA_sideslip_alphatot_phi
      | 
      | Beschreibung:
      | 
      |   Dieser Block berechnet Anstellwinkel, Schiebewinkel, totalen Anstellwinkel und Rollwinkel in [rad]
      |   aus der Geschwindigkeit vBEB (ECEF-System dargestellt in Body-Koordinaten)
      | 
      | Inputs   [dimension]  [data type] [unit]:
      | 
      |     vBEB    [3] [double] [m/s]
      | 
      | Outputs  [dimension]  [data type] [unit]:
      | 
      | aero_angle_bus [4] [bus] [-]
      |     alpha     [1] [double] [rad]
      |     beta       [1] [double] [rad]
      |     alpha_T [1] [double] [rad]
      |     phi         [1] [double] [rad]
      mask Display:
      | %port_label('input', 1, 'vBEB')
      | %port_label('output', 1, 'aero_angles')
      | disp('vBEB \rightarrow \alpha \beta \alpha_T \phi','texmode','on')
  Bus Selector : BusSelector  OutputSignals=al,be,th,fi
  Constant : Constant  Value=0.5
  Divide : Product  Inputs=*/
  Math Function1 : Math  Operator=square  SignedPower=on  SaturateOnIntegerOverflow=on
  Product1 : Product  Inputs=3
  calc_nondimensional_rates : Subsystem
  norm_of_vector : Subsystem
      mask help: computes the norm of a vector
      mask Help:
      | Name:
      | 
      |     norm_of_vector
      | 
      | Description:
      | 
      |     This block computes the L2-norm (length) of a vector.
      | 
      | Inputs  [size] [data type] [unit]:
      | 
      |     vector  [3] [double] [-]
      | 
      | Outputs  [size] [data type] [unit]:
      | 
      |     norm of vector  [1] [double] [-]
      mask Display: disp (' norm(r) ')
  al : Outport  VectorParamsAs1DForOutWhenUnconnected=off
  be : Outport  Port=2  VectorParamsAs1DForOutWhenUnconnected=off
  qdynB : Outport  Port=3  VectorParamsAs1DForOutWhenUnconnected=off
  MaB : Outport  Port=4  VectorParamsAs1DForOutWhenUnconnected=off
  a_vB : Outport  Port=5  VectorParamsAs1DForOutWhenUnconnected=off
  wBIB_star : Outport  Port=6  VectorParamsAs1DForOutWhenUnconnected=off
  th : Outport  Port=7  VectorParamsAs1DForOutWhenUnconnected=off
  fi : Outport  Port=8  VectorParamsAs1DForOutWhenUnconnected=off
  wires:
  sos/1 -> Divide/2
  AoA_Sideslip_Alphatot_Phi/1(aero_angles) -> Bus Selector/1
  vBEB/1 -> norm_of_vector/1(vector), AoA_Sideslip_Alphatot_Phi/1(vBEB)
  norm_of_vector/1(norm_of_vector) -> Math Function1/1, calc_nondimensional_rates/1(a_vB), a_vB/1, Divide/1  "a_vB"
  Product1/1 -> qdynB/1  "qdynB"
  Math Function1/1 -> Product1/1
  Constant/1 -> Product1/2
  Divide/1 -> MaB/1  "MaB"
  Bus Selector/2 -> be/1  "<be>"
  rho/1 -> Product1/3
  Bus Selector/1 -> al/1  "<al>"
  wBIB/1 -> calc_nondimensional_rates/2(wBIB)
  calc_nondimensional_rates/1(wBIB_star) -> wBIB_star/1
  Bus Selector/3 -> th/1  "<th>"
  Bus Selector/4 -> fi/1  "<fi>"
